simulink model "mFK"  (R2022b)
settings: Solver=VariableStepAuto  StartTime=0.0  StopTime=10.0  RelTol=1e-3
undefined symbols (not defined in the file): adMotorLimits
libraries: robotcorelib x1, robotmaniplib x1
settings Model: Creator=angelo  LastModifiedBy=pl130
settings DebuggingCC: UnconnectedInputMsg=warning  UnconnectedOutputMsg=warning  UnconnectedLineMsg=warning
settings ModelReferenceCC: EnableRefExpFcnMdlSchedulingChecks=on
settings RTWCC: DLArmComputeVersion=19.05

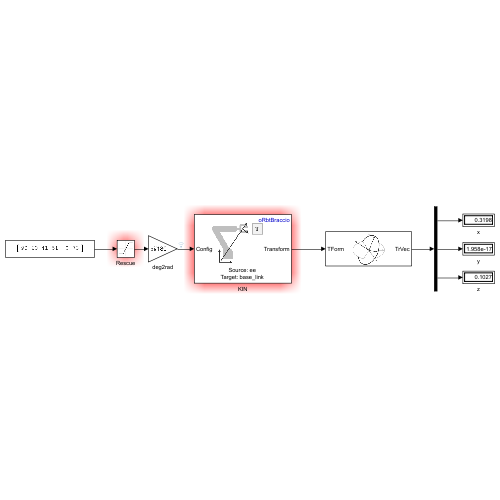
[thumbnail: Simulink's stored preview of the top-level diagram]
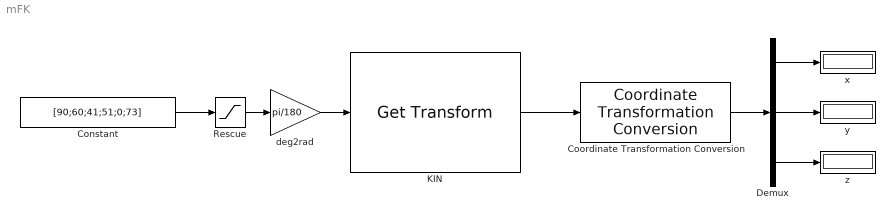
== system mFK ==
  Constant : Constant  Value=[90;60;41;51;0;73]
  Coordinate Transformation Conversion : robotcorelib/Coordinate Transformation Conversion  InputRepresentation=Homogeneous Transformation  InputEulerSequence=ZYX  ShowTrVecInputPort=on  OutputRepresentation=Translation Vector  OutputEulerSequence=ZYX  ShowTrVecOutputPort=on  SimulateUsing=Interpreted execution
  Demux : Demux  Outputs=3
  KIN : robotmaniplib/Get Transform  RigidBodyTree=oRbtBraccio  SourceBody=ee  TargetBody=base_link  SimulateUsing=Interpreted execution
  Rescue : Saturate  UpperLimit=adMotorLimits(:,2)  LowerLimit=adMotorLimits(:,1)
  deg2rad : Gain  Gain=pi/180
  x : Display
  y : Display
  z : Display
  wires:
  KIN/1 -> Coordinate Transformation Conversion/1
  Coordinate Transformation Conversion/1 -> Demux/1
  Demux/1 -> x/1
  Demux/2 -> y/1
  Demux/3 -> z/1
  Rescue/1 -> deg2rad/1
  Constant/1 -> Rescue/1
  deg2rad/1 -> KIN/1
